simulink model "Praktikum08Gruppe09"  (R2023b)
settings: Solver=VariableStepAuto  StartTime=0.0  StopTime=0.05  RelTol=1e-3
model workspace (MAT data in the model file):
  CodeRate = 0.75
  M = 16
  PunctureVector = [1; 1; 0; 1; 0; 1]
  TracebackDepth = 48
  Trelli.numInputSymbols = 2
  Trelli.numOutputSymbols = 4
  Trelli.numStates = 64
  Trelli.nextStates = [0  32; 0  32; 1  33; 1  33; 2  34; 2  34; 3  35; 3  35; 4  36; 4  36; 5  37; 5  37; 6  38; 6  38; 7  39; 7  39; 8  40; 8  40; 9  41; 9  41; 10  42; 10  42; 11  43; 11  43; 12  44; 12  44; 13  45; 13  45; 14  46; 14  46; 15  47; 15  47; 16  48; 16  48; 17  49; 17  49; 18  50; 18  50; 19  51; 19  51; 20  52; 20  52; 21  53; 21  53; 22  54; 22  54; 23  55; 23  55; 24  56; 24  56; 25  57; 25  57; 26  58; 26  58; 27  59; 27  59; 28  60; 28  60; 29  61; 29  61; 30  62; 30  62; 31  63; 31  63]
  Trelli.outputs = [0  3; 3  0; 1  2; 2  1; 0  3; 3  0; 1  2; 2  1; 3  0; 0  3; 2  1; 1  2; 3  0; 0  3; 2  1; 1  2; 3  0; 0  3; 2  1; 1  2; 3  0; 0  3; 2  1; 1  2; 0  3; 3  0; 1  2; 2  1; 0  3; 3  0; 1  2; 2  1; 2  1; 1  2; 3  0; 0  3; 2  1; 1  2; 3  0; 0  3; 1  2; 2  1; 0  3; 3  0; 1  2; 2  1; 0  3; 3  0; 1  2; 2  1; 0  3; 3  0; 1  2; 2  1; 0  3; 3  0; 2  1; 1  2; 3  0; 0  3; 2  1; 1  2; 3  0; 0  3]
  Ts = 5e-08
undefined symbols (not defined in the file): doppler, get, gray, hot, magnitude
libraries: dspstat3 x10, dspxfrm3 x8, dspobslib x7, commcnvcod2 x6, commdigbbndam3 x6, dspindex x6, commchan3 x4, commrflib2 x4, dspquant2 x4, commsink2 x4, dspsigops x4, commrandsrc3 x2
(part 1 of 2)
settings Model: Creator=suttarar@hu-berlin.de  LastModifiedBy=suttarar@hu-berlin.de

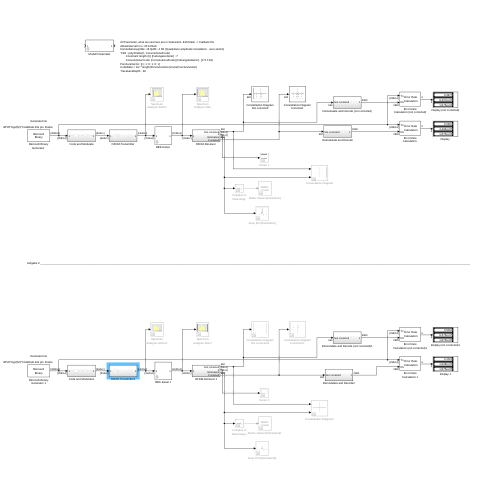
[thumbnail: Simulink's stored preview of the top-level diagram]
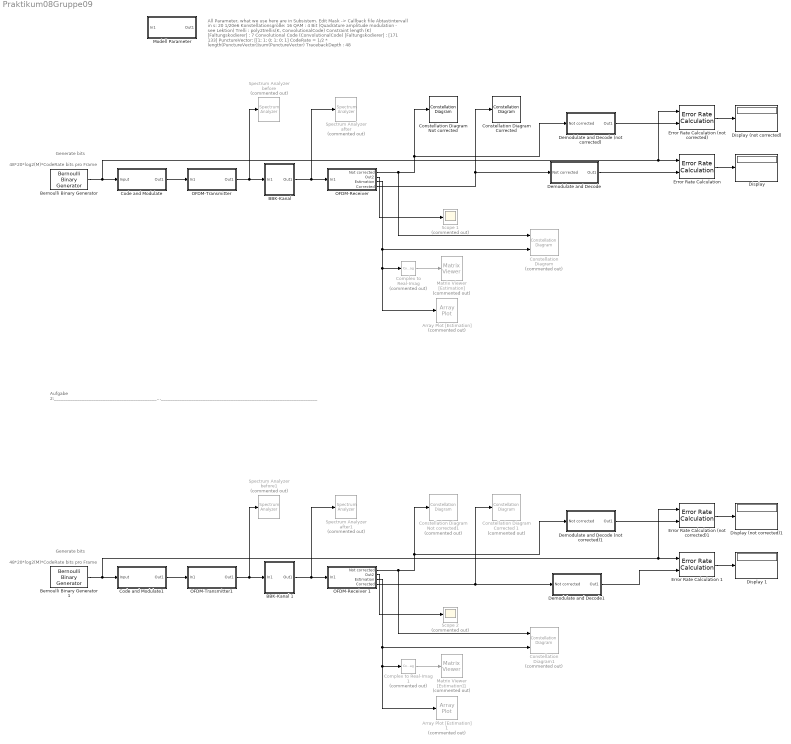
== system Praktikum08Gruppe09 ==
  note: Aufgabe 2:________________________________________________________________________________________________________________________________________________________________________________________________________________________________________________________________________________________
  note: All Parameter, what we use here are in Subsistem. Edit Mask -> Callback file
      | Abtastintervall in s: 20 1/20e6
      | Konstellationsgröße: 16 QAM : 4 Bit (Quadrature amplitude modulation - see Lektion)
      | Trelli : poly2trellis(K, ConvolutionalCode)
      | Constraint length (K) [Faltungskodierer] : 7
      | Convolutional Code (ConvolutionalCode) [Faltungskodierer] : [171 133]
      | PunctureVector: [[1; 1; 0; 1; 0; 1]
      | CodeRate = 1/2 * length(PunctureVector)/sum(PunctureVector)
      | TracebackDepth : 48
  note: 48*20*log2(M)*CodeRate bits pro Frame
  note: Generate bits
  note: 48*20*log2(M)*CodeRate bits pro Frame
  note: Generate bits
  Array Plot [Estimation] : ArrayPlot  Commented=on  WindowPosition=[886.000000,184.000000,800.000000,500.000000,]  ScopeFrameLocation=window  PlotAsMagnitudePhase=on  YLimits=[-0.4803 1.494]
  Array Plot [Estimation]1 : ArrayPlot  Commented=on  WindowPosition=[886.000000,184.000000,800.000000,500.000000,]  ScopeFrameLocation=window  PlotAsMagnitudePhase=on  YLimits=[-0.4803 1.494]
  "BBK-Kanal " : Subsystem  mask{MaxDoppler=20, PathDelays=[0 5 20].*Ts, PathGains=[0 -3 -6], EnableMultipath=1, PathLoss=0, FrequencyOffset=50, PhaseOffset=45, SNR=25}
      mask prompts: MaxDoppler "Dopplerverschiebung"; PathDelays "Pfadverzoergerungen"; PathGains "Pfadverstaerkungen"; EnableMultipath "SwitchBlock"; PathLoss "Pfadverlust"; FrequencyOffset "Frequenzverschiebung"; PhaseOffset "Phasenverschiebung"; SNR "AWG-Rauschen"
  BBK-Kanal 1 : Subsystem  mask{MaxDoppler=20, PathDelays=[0 5 20].*Ts, PathGains=[0 -3 -6], EnableMultipath=1, PathLoss=0, FrequencyOffset=50, PhaseOffset=45, SNR=25}
      mask prompts: MaxDoppler "Dopplerverschiebung"; PathDelays "Pfadverzoergerungen"; PathGains "Pfadverstaerkungen"; EnableMultipath "SwitchBlock"; PathLoss "Pfadverlust"; FrequencyOffset "Frequenzverschiebung"; PhaseOffset "Phasenverschiebung"; SNR "AWG-Rauschen"
  "Bernoulli Binary Generator " : commrandsrc3/Bernoulli Binary Generator  ProbabilityOfZero=0.5  SeedSource=Auto  Seed=0  SampleTime=Ts/(48*20*log2(M)*CodeRate)*64*24  SamplesPerFrame=48*20*log2(M)*CodeRate  OutputDataType=double  SimulateUsing=Interpreted execution
  Bernoulli Binary Generator 1 : commrandsrc3/Bernoulli Binary Generator  ProbabilityOfZero=0.5  SeedSource=Auto  Seed=0  SampleTime=Ts/(48*20*log2(M)*CodeRate)*64*24  SamplesPerFrame=48*20*log2(M)*CodeRate  OutputDataType=double  SimulateUsing=Interpreted execution
  Code and Modulate : Subsystem
  Code and Modulate1 : Subsystem
  "Complex to Real-Imag " : ComplexToRealImag  Commented=on  Output=Real
  Complex to Real-Imag 1 : ComplexToRealImag  Commented=on  Output=Real
  Constellation Diagram : ConstellationDiagram  Commented=on  NumInputPorts=2  WindowPosition=[1234.000000,143.000000,600.000000,600.000000,]  ScopeFrameLocation=window  ReferenceConstellation="{[0.70711+0.70711i        -0.70711+0.70711i        -0.70711-0.70711i         0.70711-0.70711i][0.70711+0.70711i        -0.70711+0.70711i        -0.70711-0.70711i         0.70711-0.70711i]}"  XLimits=[-1.55,1.51]  YLimits=[-1.43,1.46]  ShowLegend=on
  "Constellation Diagram Corrected " : ConstellationDiagram  WindowPosition=[121.000000,289.000000,600.000000,600.000000,]  ScopeFrameLocation=window  ReferenceConstellation="[0.70711+0.70711i        -0.70711+0.70711i        -0.70711-0.70711i         0.70711-0.70711i]"  XLimits=[-1.55,1.51]  YLimits=[-1.43,1.46]  ShowLegend=on
  Constellation Diagram Corrected 1 : ConstellationDiagram  Commented=on  WindowPosition=[121.000000,289.000000,600.000000,600.000000,]  ScopeFrameLocation=window  ReferenceConstellation="[0.70711+0.70711i        -0.70711+0.70711i        -0.70711-0.70711i         0.70711-0.70711i]"  XLimits=[-1.55,1.51]  YLimits=[-1.43,1.46]  ShowLegend=on
  Constellation Diagram Not corrected : ConstellationDiagram  WindowPosition=[922.000000,306.000000,600.000000,600.000000,]  ScopeFrameLocation=window  ReferenceConstellation="[0.70711+0.70711i        -0.70711+0.70711i        -0.70711-0.70711i         0.70711-0.70711i]"  XLimits=[-1.55,1.51]  YLimits=[-1.43,1.46]  ShowLegend=on
  Constellation Diagram Not corrected1 : ConstellationDiagram  Commented=on  WindowPosition=[922.000000,306.000000,600.000000,600.000000,]  ScopeFrameLocation=window  ReferenceConstellation="[0.70711+0.70711i        -0.70711+0.70711i        -0.70711-0.70711i         0.70711-0.70711i]"  XLimits=[-1.55,1.51]  YLimits=[-1.43,1.46]  ShowLegend=on
  Constellation Diagram1 : ConstellationDiagram  Commented=on  NumInputPorts=2  WindowPosition=[1234.000000,143.000000,600.000000,600.000000,]  ScopeFrameLocation=window  ReferenceConstellation="{[0.70711+0.70711i        -0.70711+0.70711i        -0.70711-0.70711i         0.70711-0.70711i][0.70711+0.70711i        -0.70711+0.70711i        -0.70711-0.70711i         0.70711-0.70711i]}"  XLimits=[-1.55,1.51]  YLimits=[-1.43,1.46]  ShowLegend=on
  Demodulate and Decode : Subsystem
  Demodulate and Decode (not corrected) : Subsystem
  Demodulate and Decode (not corrected)1 : Subsystem
  Demodulate and Decode1 : Subsystem
  "Display " : Display
  Display (not corrected) : Display
  Display (not corrected)1 : Display
  Display 1 : Display
  "Error Rate Calculation " : commsink2/Error Rate Calculation  N=TracebackDepth  st_delay=48*20*log2(M)*CodeRate  cp_mode=Entire frame  subframe=[]  PMode=Port  WsName=ErrorVec  RsMode2=off  stop=off  numErr=100  maxBits=1e6
  Error Rate Calculation (not corrected) : commsink2/Error Rate Calculation  N=TracebackDepth  st_delay=48*20*log2(M)*CodeRate  cp_mode=Entire frame  subframe=[]  PMode=Port  WsName=ErrorVec  RsMode2=off  stop=off  numErr=100  maxBits=1e6
  Error Rate Calculation (not corrected)1 : commsink2/Error Rate Calculation  N=TracebackDepth  st_delay=48*20*log2(M)*CodeRate  cp_mode=Entire frame  subframe=[]  PMode=Port  WsName=ErrorVec  RsMode2=off  stop=off  numErr=100  maxBits=1e6
  Error Rate Calculation 1 : commsink2/Error Rate Calculation  N=TracebackDepth  st_delay=48*20*log2(M)*CodeRate  cp_mode=Entire frame  subframe=[]  PMode=Port  WsName=ErrorVec  RsMode2=off  stop=off  numErr=100  maxBits=1e6
  Matrix Viewer [Estimation] : dspobslib/Matrix Viewer  Commented=on  ImageParams=off  CMapStr=gray(256)  AxisColorbar=on  AxisParams=off  AxisOrigin=Upper left corner  AxisTickMode=Auto  XTickRange=[0 1]  YTickRange=[0 1]  XLabel=X-axis  YLabel=Y-axis  ZLabel=Z-axis  FigPos=get(0,'defaultfigureposition')  AxisZoom=off
      settings: YMin=0.99546  YMax=1.0044
  Matrix Viewer [Estimation]1 : dspobslib/Matrix Viewer  Commented=on  ImageParams=off  CMapStr=gray(256)  AxisColorbar=on  AxisParams=off  AxisOrigin=Upper left corner  AxisTickMode=Auto  XTickRange=[0 1]  YTickRange=[0 1]  XLabel=X-axis  YLabel=Y-axis  ZLabel=Z-axis  FigPos=get(0,'defaultfigureposition')  AxisZoom=off
      settings: YMin=0.99546  YMax=1.0044
  Modell Parameter : Subsystem  mask{Ts=1/20e6, M=16, Trelli=poly2trellis(7, [171 133]), PunctureVector=[1; 1; 0; 1; 0; 1], CodeRate=0.75, TracebackDepth=48}
      mask prompts: Ts "Abtastintervall in s"; M "Konstellationsgröße"
  "OFDM-Receiver " : Subsystem
  OFDM-Receiver 1 : Subsystem
  OFDM-Transmitter : Subsystem
  OFDM-Transmitter1 : Subsystem
  Scope 1 : Scope  Commented=on
  Scope 2 : Scope  Commented=on
  Spectrum Analyzer after : SpectrumAnalyzer  Commented=on  WindowPosition=[-15.000000,19.000000,800.000000,500.000000,]  ScopeFrameLocation=window  Span=20000000  StartFrequency=-10000000  StopFrequency=10000000  YLimits=[-31.57647303,17.61555358]
  Spectrum Analyzer after1 : SpectrumAnalyzer  Commented=on  WindowPosition=[-15.000000,19.000000,800.000000,500.000000,]  ScopeFrameLocation=window  Span=20000000  StartFrequency=-10000000  StopFrequency=10000000  YLimits=[-31.57647303,17.61555358]
  Spectrum Analyzer before : SpectrumAnalyzer  Commented=on  WindowPosition=[6.000000,502.000000,800.000000,500.000000,]  ScopeFrameLocation=window  Span=20000000  StartFrequency=-10000000  StopFrequency=10000000  YLimits=[-48.78355479,20.07673212]
  Spectrum Analyzer before1 : SpectrumAnalyzer  Commented=on  WindowPosition=[6.000000,502.000000,800.000000,500.000000,]  ScopeFrameLocation=window  Span=20000000  StartFrequency=-10000000  StopFrequency=10000000  YLimits=[-48.78355479,20.07673212]
  wires:
  Code and Modulate/1(Out1) -> OFDM-Transmitter/1(In1)
  "OFDM-Receiver "/2(Out2) -> Scope 1/1
  "BBK-Kanal "/1(Out1) -> Spectrum Analyzer after/1, "OFDM-Receiver "/1(In1)
  OFDM-Transmitter/1(Out1) -> Spectrum Analyzer before/1, "BBK-Kanal "/1(In1)
  "OFDM-Receiver "/1(Not corrected) -> Demodulate and Decode (not corrected)/1(Not corrected), Constellation Diagram Not corrected/1, Constellation Diagram/1
  "Error Rate Calculation "/1 -> "Display "/1
  "Bernoulli Binary Generator "/1 -> Error Rate Calculation (not corrected)/1, "Error Rate Calculation "/1, Code and Modulate/1(Input)
  "Complex to Real-Imag "/1 -> Matrix Viewer [Estimation]/1
  "OFDM-Receiver "/3(Estimation) -> Constellation Diagram/2, Array Plot [Estimation]/1, "Complex to Real-Imag "/1
  Demodulate and Decode/1(Out1) -> "Error Rate Calculation "/2
  "OFDM-Receiver "/4(Corrected) -> Demodulate and Decode/1(Not corrected), "Constellation Diagram Corrected "/1
  Error Rate Calculation (not corrected)/1 -> Display (not corrected)/1
  Demodulate and Decode (not corrected)/1(Out1) -> Error Rate Calculation (not corrected)/2
  OFDM-Receiver 1/1(Not corrected) -> Demodulate and Decode (not corrected)1/1(Not corrected), Constellation Diagram Not corrected1/1, Constellation Diagram1/1
  Code and Modulate1/1(Out1) -> OFDM-Transmitter1/1(In1)
  Complex to Real-Imag 1/1 -> Matrix Viewer [Estimation]1/1
  BBK-Kanal 1/1(Out1) -> Spectrum Analyzer after1/1, OFDM-Receiver 1/1(In1)
  OFDM-Receiver 1/2(Out2) -> Scope 2/1
  OFDM-Receiver 1/4(Corrected) -> Constellation Diagram Corrected 1/1, Demodulate and Decode1/1(Not corrected)
  Error Rate Calculation 1/1 -> Display 1/1
  Error Rate Calculation (not corrected)1/1 -> Display (not corrected)1/1
  Demodulate and Decode (not corrected)1/1(Out1) -> Error Rate Calculation (not corrected)1/2
  OFDM-Transmitter1/1(Out1) -> Spectrum Analyzer before1/1, BBK-Kanal 1/1(In1)
  Demodulate and Decode1/1(Out1) -> Error Rate Calculation 1/2
  Bernoulli Binary Generator 1/1 -> Error Rate Calculation (not corrected)1/1, Error Rate Calculation 1/1, Code and Modulate1/1(Input)
  OFDM-Receiver 1/3(Estimation) -> Constellation Diagram1/2, Array Plot [Estimation]1/1, Complex to Real-Imag 1/1

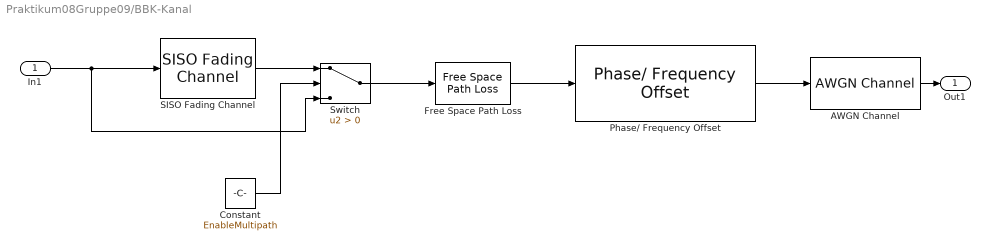
== system Praktikum08Gruppe09/BBK-Kanal  ==
  In1 : Inport
  AWGN Channel : commchan3/AWGN Channel  LegacyMode=off  NoiseMethod="Signal to noise ratio  (SNR)"  noiseMode="Signal to noise ratio  (SNR)"  EbNo=10  EsNo=10  SNR=SNR  BitsPerSymbol=1  SignalPower=1  SamplesPerSymbol=1  SymbolPeriod=1  VarianceSource=Parameter  Variance=1  RandomStream=Global stream  Seed=67  SimulateUsing=Code generation
  Constant : Constant  Value=EnableMultipath
  Free Space Path Loss : commrflib2/Free Space Path Loss  mode=Decibels  dB=PathLoss  d=0.100  fc=1920
  Phase/ Frequency Offset : commrflib2/Phase// Frequency Offset  phaseOffset=PhaseOffset  freqPort=off  freqOffset=FrequencyOffset
      settings: LibrarySourceBlock=|
      | commrfcorlib/Phase//
      | Frequency
      | Offset
  SISO Fading Channel : commchan3/SISO Fading Channel  InheritSampleRate=on  SampleRate=1  PathDelays=PathDelays  AveragePathGains=PathGains  NormalizePathGains=on  FadingDistribution=Rayleigh  KFactor=3  DirectPathDopplerShift=0  DirectPathInitialPhase=0  MaximumDopplerShift=MaxDoppler  DopplerSpectrum=doppler('Jakes')  RandomStream=mt19937ar with seed  Seed=73  PathGainsOutputPort=off  ChannelFilterDelayOutputPort=off  SimulateUsing=Interpreted execution  Visualization=Off  PathsForDopplerDisplay=1  SamplesToDisplay=25%
  Switch : Switch  Criteria=u2 > Threshold  SaturateOnIntegerOverflow=off  InputSameDT=off
  Out1 : Outport
  wires:
  Phase/ Frequency Offset/1 -> AWGN Channel/1
  Free Space Path Loss/1 -> Phase/ Frequency Offset/1
  AWGN Channel/1 -> Out1/1
  Switch/1 -> Free Space Path Loss/1
  SISO Fading Channel/1 -> Switch/1
  In1/1 -> Switch/3, SISO Fading Channel/1
  Constant/1 -> Switch/2

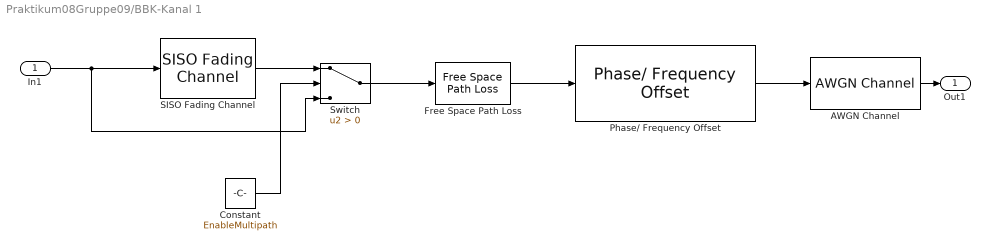
== system Praktikum08Gruppe09/BBK-Kanal 1 ==
  In1 : Inport
  AWGN Channel : commchan3/AWGN Channel  LegacyMode=off  NoiseMethod="Signal to noise ratio  (SNR)"  noiseMode="Signal to noise ratio  (SNR)"  EbNo=10  EsNo=10  SNR=SNR  BitsPerSymbol=1  SignalPower=1  SamplesPerSymbol=1  SymbolPeriod=1  VarianceSource=Parameter  Variance=1  RandomStream=Global stream  Seed=67  SimulateUsing=Code generation
  Constant : Constant  Value=EnableMultipath
  Free Space Path Loss : commrflib2/Free Space Path Loss  mode=Decibels  dB=PathLoss  d=0.100  fc=1920
  Phase/ Frequency Offset : commrflib2/Phase// Frequency Offset  phaseOffset=PhaseOffset  freqPort=off  freqOffset=FrequencyOffset
      settings: LibrarySourceBlock=|
      | commrfcorlib/Phase//
      | Frequency
      | Offset
  SISO Fading Channel : commchan3/SISO Fading Channel  InheritSampleRate=on  SampleRate=1  PathDelays=PathDelays  AveragePathGains=PathGains  NormalizePathGains=on  FadingDistribution=Rayleigh  KFactor=3  DirectPathDopplerShift=0  DirectPathInitialPhase=0  MaximumDopplerShift=MaxDoppler  DopplerSpectrum=doppler('Jakes')  RandomStream=mt19937ar with seed  Seed=73  PathGainsOutputPort=off  ChannelFilterDelayOutputPort=off  SimulateUsing=Interpreted execution  Visualization=Off  PathsForDopplerDisplay=1  SamplesToDisplay=25%
  Switch : Switch  Criteria=u2 > Threshold  SaturateOnIntegerOverflow=off  InputSameDT=off
  Out1 : Outport
  wires:
  Phase/ Frequency Offset/1 -> AWGN Channel/1
  Free Space Path Loss/1 -> Phase/ Frequency Offset/1
  AWGN Channel/1 -> Out1/1
  Switch/1 -> Free Space Path Loss/1
  SISO Fading Channel/1 -> Switch/1
  In1/1 -> Switch/3, SISO Fading Channel/1
  Constant/1 -> Switch/2

== system Praktikum08Gruppe09/Code and Modulate ==
  note: Modulation
  note: Faltungscodierer
  Input : Inport
  "Convolutional Encoder " : commcnvcod2/Convolutional Encoder  trellis=Trelli  opMode=Continuous  DelayedResetAction=off  hasIniStPort=off  hasFinStPort=off  usePuncVector=on  punctureVector=PunctureVector  reset=Unused parameter value
  "Rectangular QAM Modulator Baseband " : commdigbbndam3/Rectangular QAM Modulator Baseband  M=M  InType=Bit  Enc=Gray  Mapping=[0:15]  PowType=Average Power  MinDist=2  AvgPow=1  PeakPow=1  Ph=0  outDtype=double  outWordLen=16  outUDDataType=sfix(16)  outFracLenMode=Best precision  outFracLen=15  outDataTypeStr=double  outLastDataTypeStr=double
  Out1 : Outport
  wires:
  "Convolutional Encoder "/1 -> "Rectangular QAM Modulator Baseband "/1
  "Rectangular QAM Modulator Baseband "/1 -> Out1/1
  Input/1 -> "Convolutional Encoder "/1

== system Praktikum08Gruppe09/Code and Modulate1 ==
  note: Modulation
  note: Faltungscodierer
  Input : Inport
  "Convolutional Encoder " : commcnvcod2/Convolutional Encoder  trellis=Trelli  opMode=Continuous  DelayedResetAction=off  hasIniStPort=off  hasFinStPort=off  usePuncVector=on  punctureVector=PunctureVector  reset=Unused parameter value
  "Rectangular QAM Modulator Baseband " : commdigbbndam3/Rectangular QAM Modulator Baseband  M=M  InType=Bit  Enc=Gray  Mapping=[0:15]  PowType=Average Power  MinDist=2  AvgPow=1  PeakPow=1  Ph=0  outDtype=double  outWordLen=16  outUDDataType=sfix(16)  outFracLenMode=Best precision  outFracLen=15  outDataTypeStr=double  outLastDataTypeStr=double
  Out1 : Outport
  wires:
  "Convolutional Encoder "/1 -> "Rectangular QAM Modulator Baseband "/1
  "Rectangular QAM Modulator Baseband "/1 -> Out1/1
  Input/1 -> "Convolutional Encoder "/1

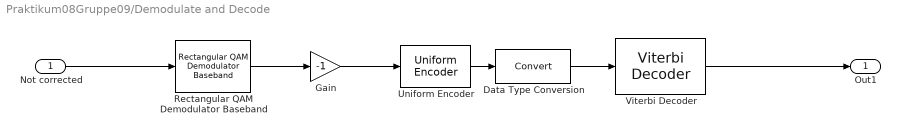
== system Praktikum08Gruppe09/Demodulate and Decode ==
  Not corrected : Inport
  "Data Type Conversion " : DataTypeConversion  SaturateOnIntegerOverflow=off  RndMeth=Floor
  "Gain " : Gain  Gain=-1
  "Rectangular QAM Demodulator Baseband " : commdigbbndam3/Rectangular QAM Demodulator Baseband  M=M  OutType=Bit  DecType=Approximate log-likelihood ratio  VarSource=Dialog  Variance=1  Dec=Gray  Mapping=[0:15]  PowType=Average Power  MinDist=2  AvgPow=1  PeakPow=1  Ph=0  outDtype1=Inherit via internal rule  outDtype2=Inherit via internal rule  derotateFactorWordLen=16  derotateFactorDataTypeStr=Inherit: Same word length as input  derotateFactorLastDataTypeStr=Inherit: Same word length as input  denormFactorWordLen=16  denormFactorDataTypeStr=Inherit: Same word length as input  denormFactorLastDataTypeStr=Inherit: Same word length as input  prodOutWordLen=32  prodOutOverflowMode=Wrap  prodOutRoundingMode=Floor  prodOutOvFlMode=off  prodOutOvFlModeLastStrValue=off  sumWordLen=32
  "Uniform Encoder " : dspquant2/Uniform Encoder  peak=1  bits=4  otype=Unsigned integer
  "Viterbi Decoder " : commcnvcod2/Viterbi Decoder  trellis=Trelli  isPunctured=on  punctureVector=PunctureVector  erasures=off  dectype=Soft decision  nsdecb=4  runSigValErrCheck=off  tbdepth=TracebackDepth  opmode=Continuous  reset=off  delayedResetAction=off  smWordLength=16  outDataType=double
  Out1 : Outport
  wires:
  "Uniform Encoder "/1 -> "Data Type Conversion "/1
  "Gain "/1 -> "Uniform Encoder "/1
  "Data Type Conversion "/1 -> "Viterbi Decoder "/1
  "Rectangular QAM Demodulator Baseband "/1 -> "Gain "/1
  Not corrected/1 -> "Rectangular QAM Demodulator Baseband "/1
  "Viterbi Decoder "/1 -> Out1/1

== system Praktikum08Gruppe09/Demodulate and Decode (not corrected) ==
  Not corrected : Inport
  "Data Type Conversion " : DataTypeConversion  SaturateOnIntegerOverflow=off  RndMeth=Floor
  "Gain " : Gain  Gain=-1
  "Rectangular QAM Demodulator Baseband " : commdigbbndam3/Rectangular QAM Demodulator Baseband  M=M  OutType=Bit  DecType=Approximate log-likelihood ratio  VarSource=Dialog  Variance=1  Dec=Gray  Mapping=[0:15]  PowType=Average Power  MinDist=2  AvgPow=1  PeakPow=1  Ph=0  outDtype1=Inherit via internal rule  outDtype2=Inherit via internal rule  derotateFactorWordLen=16  derotateFactorDataTypeStr=Inherit: Same word length as input  derotateFactorLastDataTypeStr=Inherit: Same word length as input  denormFactorWordLen=16  denormFactorDataTypeStr=Inherit: Same word length as input  denormFactorLastDataTypeStr=Inherit: Same word length as input  prodOutWordLen=32  prodOutOverflowMode=Wrap  prodOutRoundingMode=Floor  prodOutOvFlMode=off  prodOutOvFlModeLastStrValue=off  sumWordLen=32
  "Uniform Encoder " : dspquant2/Uniform Encoder  peak=1  bits=4  otype=Unsigned integer
  "Viterbi Decoder " : commcnvcod2/Viterbi Decoder  trellis=Trelli  isPunctured=on  punctureVector=PunctureVector  erasures=off  dectype=Soft decision  nsdecb=4  runSigValErrCheck=off  tbdepth=TracebackDepth  opmode=Continuous  reset=off  delayedResetAction=off  smWordLength=16  outDataType=double
  Out1 : Outport
  wires:
  "Uniform Encoder "/1 -> "Data Type Conversion "/1
  "Gain "/1 -> "Uniform Encoder "/1
  "Data Type Conversion "/1 -> "Viterbi Decoder "/1
  "Rectangular QAM Demodulator Baseband "/1 -> "Gain "/1
  Not corrected/1 -> "Rectangular QAM Demodulator Baseband "/1
  "Viterbi Decoder "/1 -> Out1/1

== system Praktikum08Gruppe09/Demodulate and Decode (not corrected)1 ==
  Not corrected : Inport
  "Data Type Conversion " : DataTypeConversion  SaturateOnIntegerOverflow=off  RndMeth=Floor
  "Gain " : Gain  Gain=-1
  "Rectangular QAM Demodulator Baseband " : commdigbbndam3/Rectangular QAM Demodulator Baseband  M=M  OutType=Bit  DecType=Approximate log-likelihood ratio  VarSource=Dialog  Variance=1  Dec=Gray  Mapping=[0:15]  PowType=Average Power  MinDist=2  AvgPow=1  PeakPow=1  Ph=0  outDtype1=Inherit via internal rule  outDtype2=Inherit via internal rule  derotateFactorWordLen=16  derotateFactorDataTypeStr=Inherit: Same word length as input  derotateFactorLastDataTypeStr=Inherit: Same word length as input  denormFactorWordLen=16  denormFactorDataTypeStr=Inherit: Same word length as input  denormFactorLastDataTypeStr=Inherit: Same word length as input  prodOutWordLen=32  prodOutOverflowMode=Wrap  prodOutRoundingMode=Floor  prodOutOvFlMode=off  prodOutOvFlModeLastStrValue=off  sumWordLen=32
  "Uniform Encoder " : dspquant2/Uniform Encoder  peak=1  bits=4  otype=Unsigned integer
  "Viterbi Decoder " : commcnvcod2/Viterbi Decoder  trellis=Trelli  isPunctured=on  punctureVector=PunctureVector  erasures=off  dectype=Soft decision  nsdecb=4  runSigValErrCheck=off  tbdepth=TracebackDepth  opmode=Continuous  reset=off  delayedResetAction=off  smWordLength=16  outDataType=double
  Out1 : Outport
  wires:
  "Uniform Encoder "/1 -> "Data Type Conversion "/1
  "Gain "/1 -> "Uniform Encoder "/1
  "Data Type Conversion "/1 -> "Viterbi Decoder "/1
  "Rectangular QAM Demodulator Baseband "/1 -> "Gain "/1
  Not corrected/1 -> "Rectangular QAM Demodulator Baseband "/1
  "Viterbi Decoder "/1 -> Out1/1

== system Praktikum08Gruppe09/Demodulate and Decode1 ==
  Not corrected : Inport
  "Data Type Conversion " : DataTypeConversion  SaturateOnIntegerOverflow=off  RndMeth=Floor
  "Gain " : Gain  Gain=-1
  "Rectangular QAM Demodulator Baseband " : commdigbbndam3/Rectangular QAM Demodulator Baseband  M=M  OutType=Bit  DecType=Approximate log-likelihood ratio  VarSource=Dialog  Variance=1  Dec=Gray  Mapping=[0:15]  PowType=Average Power  MinDist=2  AvgPow=1  PeakPow=1  Ph=0  outDtype1=Inherit via internal rule  outDtype2=Inherit via internal rule  derotateFactorWordLen=16  derotateFactorDataTypeStr=Inherit: Same word length as input  derotateFactorLastDataTypeStr=Inherit: Same word length as input  denormFactorWordLen=16  denormFactorDataTypeStr=Inherit: Same word length as input  denormFactorLastDataTypeStr=Inherit: Same word length as input  prodOutWordLen=32  prodOutOverflowMode=Wrap  prodOutRoundingMode=Floor  prodOutOvFlMode=off  prodOutOvFlModeLastStrValue=off  sumWordLen=32
  "Uniform Encoder " : dspquant2/Uniform Encoder  peak=1  bits=4  otype=Unsigned integer
  "Viterbi Decoder " : commcnvcod2/Viterbi Decoder  trellis=Trelli  isPunctured=on  punctureVector=PunctureVector  erasures=off  dectype=Soft decision  nsdecb=4  runSigValErrCheck=off  tbdepth=TracebackDepth  opmode=Continuous  reset=off  delayedResetAction=off  smWordLength=16  outDataType=double
  Out1 : Outport
  wires:
  "Uniform Encoder "/1 -> "Data Type Conversion "/1
  "Gain "/1 -> "Uniform Encoder "/1
  "Data Type Conversion "/1 -> "Viterbi Decoder "/1
  "Rectangular QAM Demodulator Baseband "/1 -> "Gain "/1
  Not corrected/1 -> "Rectangular QAM Demodulator Baseband "/1
  "Viterbi Decoder "/1 -> Out1/1

== system Praktikum08Gruppe09/Modell Parameter ==
  In1 : Inport
  Out1 : Outport
  wires:
  In1/1 -> Out1/1

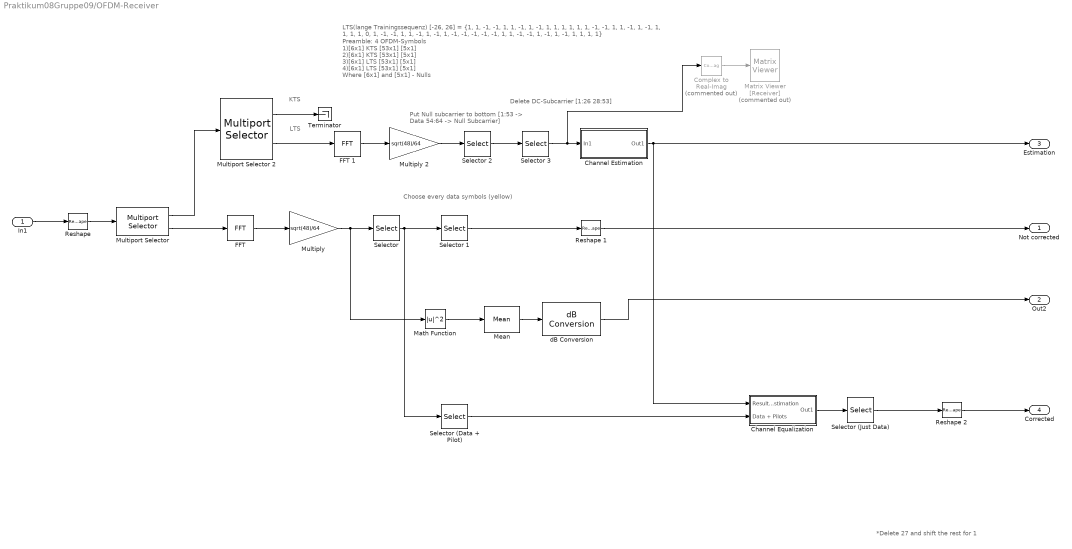
== system Praktikum08Gruppe09/OFDM-Receiver  ==
  note: *Delete 27 and shift the rest for 1
  note: Delete DC-Subcarrier [1:26 28:53]
  note: Put Null subcarrier to bottom
      | [1:53 -> Data 54:64 -> Null Subcarrier]
  note: LTS
  note: KTS
  note: Choose every data symbols (yellow)
  note: LTS(lange Trainingssequenz) [-26, 26] = {1, 1, -1, -1, 1, 1, -1, 1, -1, 1, 1, 1, 1, 1, 1, -1, -1, 1, 1, -1, 1, -1, 1, 1, 1, 1, 0, 1, -1, -1, 1, 1, -1, 1, -1, 1, -1, -1, -1, -1, -1, 1, 1, -1, -1, 1, -1, 1, -1, 1, 1, 1, 1}
  note: Preamble: 4 OFDM-Symbols
      | 1)[6x1] KTS [53x1] [5x1]
      | 2)[6x1] KTS [53x1] [5x1]
      | 3)[6x1] LTS [53x1] [5x1]
      | 4)[6x1] LTS [53x1] [5x1]
      |
      | Where [6x1] and [5x1] - Nulls
  In1 : Inport
  Channel Equalization : Subsystem
  Channel Estimation : Subsystem
  "Complex to Real-Imag " : ComplexToRealImag  Commented=on  Output=Real
  "FFT " : dspxfrm3/FFT  FFTImplementation=Auto  CompMethod=Table lookup  TableOpt=NEW  TableOptActive=Speed  BitRevOrder=off  Normalize=off  InheritFFTLength=on  FFTLength=64  WrapInput=on  roundingMode=Floor  overflowMode=off  firstCoeffDataTypeStr=Inherit: Same word length as input  firstCoeffLastDataTypeStr=Inherit: Same word length as input  outputMin=[]  outputMax=[]
  FFT 1 : dspxfrm3/FFT  FFTImplementation=Auto  CompMethod=Table lookup  TableOpt=NEW  TableOptActive=Speed  BitRevOrder=off  Normalize=off  InheritFFTLength=on  FFTLength=64  WrapInput=on  roundingMode=Floor  overflowMode=off  firstCoeffDataTypeStr=Inherit: Same word length as input  firstCoeffLastDataTypeStr=Inherit: Same word length as input  outputMin=[]  outputMax=[]
  "Math Function " : Math  Operator=magnitude^2
  Matrix Viewer [Receiver] : dspobslib/Matrix Viewer  Commented=on  ImageParams=off  CMapStr=gray(256)  AxisColorbar=on  AxisParams=off  AxisOrigin=Upper left corner  AxisTickMode=Auto  XTickRange=[0 1]  YTickRange=[0 1]  XLabel=X-axis  YLabel=Y-axis  ZLabel=Z-axis  FigPos=get(0,'defaultfigureposition')  AxisZoom=off
      settings: YMin=-1.0038  YMax=1.0044
  "Mean " : dspstat3/Mean  run=off  InputProcessing=Columns as channels (frame based)  reset_popup=None  directionMode=Each row  dimension=1  roiEnable=off  roiType=Rectangles  roiPortion=Entire ROI  roiOutput=Individual statistics for each ROI  roiFlag=off  roundingMode=Floor  overflowMode=off  outputDataTypeStr=Inherit: Same as accumulator  outputMin=[]  outputMax=[]  outputLastDataTypeStr=Inherit: Same as accumulator
  "Multiply " : Gain  Gain=sqrt(48)/64
  Multiply 2 : Gain  Gain=sqrt(48)/64
  "Multiport Selector " : dspindex/Multiport Selector  rowsOrCols=Columns  idxCellArray={[1:4], [5:24]}  idxErrMode=Clip Index
  Multiport Selector 2 : dspindex/Multiport Selector  rowsOrCols=Columns  idxCellArray={[1:2], [3:4]}  idxErrMode=Clip Index
  "Reshape " : Reshape  OutputDimensionality=Customize  OutputDimensions=[64,24]
  Reshape 1 : Reshape  OutputDimensions=[64,24]
  Reshape 2 : Reshape  OutputDimensions=[64,24]
  "Selector " : Selector  NumberOfDimensions=2  InputPortWidth=3  IndexOptions=Index vector (dialog),Select all  Indices=[39:64 1:38],1  OutputSizes=1,1
  Selector (Data + Pilot) : Selector  NumberOfDimensions=2  InputPortWidth=3  IndexOptions=Index vector (dialog),Select all  Indices=[1:26 28:53],1  OutputSizes=1,1
  Selector (Just Data) : Selector  NumberOfDimensions=2  InputPortWidth=3  IndexOptions=Index vector (dialog),Select all  Indices=[1:5 7:19 21:32 34:46 48:52],1  OutputSizes=1,1
  Selector 1 : Selector  NumberOfDimensions=2  InputPortWidth=3  IndexOptions=Index vector (dialog),Select all  Indices=[1:5 7:19 21:26 28:33 35:47 49:53],1  OutputSizes=1,1
  Selector 2 : Selector  NumberOfDimensions=2  InputPortWidth=3  IndexOptions=Index vector (dialog),Select all  Indices=[39:64 1:38],1  OutputSizes=1,1
  Selector 3 : Selector  NumberOfDimensions=2  InputPortWidth=3  IndexOptions=Index vector (dialog),Select all  Indices=[1:26 28:53],1  OutputSizes=1,1
  "Terminator " : Terminator
  "dB Conversion " : dspmathops/dB Conversion  dBtype=dB  intype=Power  R=1  fuzz=off
      settings: LibrarySourceBlock=commutil2/dB Conversion
  Not corrected : Outport
  Out2 : Outport  Port=2
  Estimation : Outport  Port=3
  Corrected : Outport  Port=4
  wires:
  "Mean "/1 -> "dB Conversion "/1
  "Math Function "/1 -> "Mean "/1
  "FFT "/1 -> "Multiply "/1
  In1/1 -> "Reshape "/1
  "Selector "/1 -> Selector (Data + Pilot)/1, Selector 1/1
  "Reshape "/1 -> "Multiport Selector "/1
  "Multiport Selector "/2 -> "FFT "/1
  "Multiport Selector "/1 -> Multiport Selector 2/1
  "dB Conversion "/1 -> Out2/1
  Selector 1/1 -> Reshape 1/1
  Reshape 1/1 -> Not corrected/1
  "Multiply "/1 -> "Math Function "/1, "Selector "/1
  Multiport Selector 2/1 -> "Terminator "/1
  Multiport Selector 2/2 -> FFT 1/1
  Channel Estimation/1(Out1) -> Channel Equalization/1(Result from Channel Estimation), Estimation/1
  Selector 2/1 -> Selector 3/1
  Multiply 2/1 -> Selector 2/1
  FFT 1/1 -> Multiply 2/1
  Selector 3/1 -> "Complex to Real-Imag "/1, Channel Estimation/1(In1)
  "Complex to Real-Imag "/1 -> Matrix Viewer [Receiver]/1
  Selector (Data + Pilot)/1 -> Channel Equalization/2(Data + Pilots)
  Channel Equalization/1(Out1) -> Selector (Just Data)/1
  Selector (Just Data)/1 -> Reshape 2/1
  Reshape 2/1 -> Corrected/1

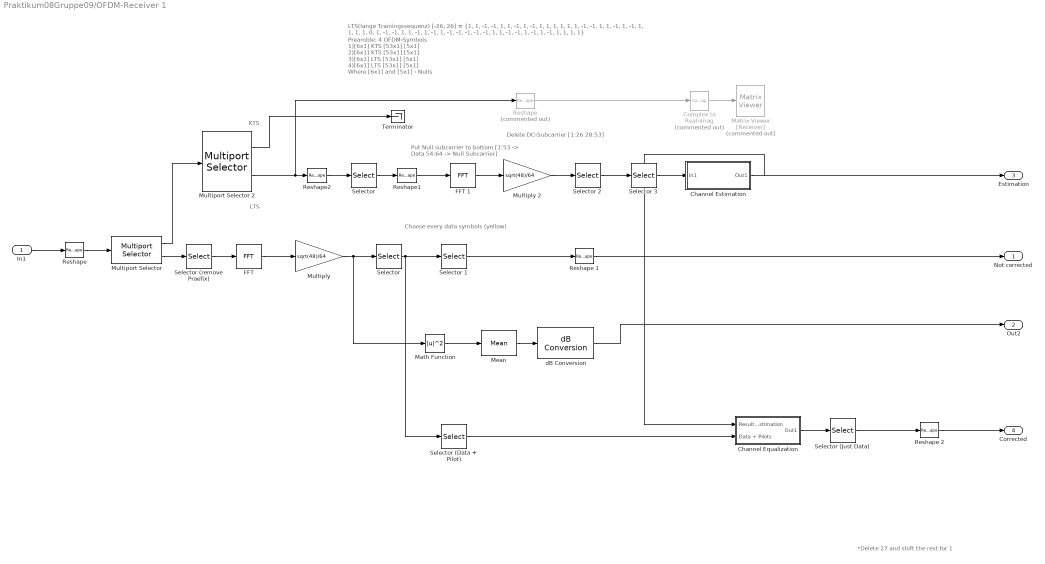
== system Praktikum08Gruppe09/OFDM-Receiver 1 ==
  note: *Delete 27 and shift the rest for 1
  note: Delete DC-Subcarrier [1:26 28:53]
  note: Put Null subcarrier to bottom
      | [1:53 -> Data 54:64 -> Null Subcarrier]
  note: LTS
  note: KTS
  note: Choose every data symbols (yellow)
  note: LTS(lange Trainingssequenz) [-26, 26] = {1, 1, -1, -1, 1, 1, -1, 1, -1, 1, 1, 1, 1, 1, 1, -1, -1, 1, 1, -1, 1, -1, 1, 1, 1, 1, 0, 1, -1, -1, 1, 1, -1, 1, -1, 1, -1, -1, -1, -1, -1, 1, 1, -1, -1, 1, -1, 1, -1, 1, 1, 1, 1}
  note: Preamble: 4 OFDM-Symbols
      | 1)[6x1] KTS [53x1] [5x1]
      | 2)[6x1] KTS [53x1] [5x1]
      | 3)[6x1] LTS [53x1] [5x1]
      | 4)[6x1] LTS [53x1] [5x1]
      |
      | Where [6x1] and [5x1] - Nulls
  In1 : Inport
  Channel Equalization : Subsystem
  Channel Estimation : Subsystem
  "Complex to Real-Imag " : ComplexToRealImag  Commented=on  Output=Real
  "FFT " : dspxfrm3/FFT  FFTImplementation=Auto  CompMethod=Table lookup  TableOpt=NEW  TableOptActive=Speed  BitRevOrder=off  Normalize=off  InheritFFTLength=on  FFTLength=64  WrapInput=on  roundingMode=Floor  overflowMode=off  firstCoeffDataTypeStr=Inherit: Same word length as input  firstCoeffLastDataTypeStr=Inherit: Same word length as input  outputMin=[]  outputMax=[]
  FFT 1 : dspxfrm3/FFT  FFTImplementation=Auto  CompMethod=Table lookup  TableOpt=NEW  TableOptActive=Speed  BitRevOrder=off  Normalize=off  InheritFFTLength=on  FFTLength=64  WrapInput=on  roundingMode=Floor  overflowMode=off  firstCoeffDataTypeStr=Inherit: Same word length as input  firstCoeffLastDataTypeStr=Inherit: Same word length as input  outputMin=[]  outputMax=[]
  "Math Function " : Math  Operator=magnitude^2
  Matrix Viewer [Receiver] : dspobslib/Matrix Viewer  Commented=on  ImageParams=off  CMapStr=gray(256)  AxisColorbar=on  AxisParams=off  AxisOrigin=Upper left corner  AxisTickMode=Auto  XTickRange=[0 1]  YTickRange=[0 1]  XLabel=X-axis  YLabel=Y-axis  ZLabel=Z-axis  FigPos=get(0,'defaultfigureposition')  AxisZoom=off
      settings: YMin=-1.4434  YMax=1.4434
  "Mean " : dspstat3/Mean  run=off  InputProcessing=Columns as channels (frame based)  reset_popup=None  directionMode=Each row  dimension=1  roiEnable=off  roiType=Rectangles  roiPortion=Entire ROI  roiOutput=Individual statistics for each ROI  roiFlag=off  roundingMode=Floor  overflowMode=off  outputDataTypeStr=Inherit: Same as accumulator  outputMin=[]  outputMax=[]  outputLastDataTypeStr=Inherit: Same as accumulator
  "Multiply " : Gain  Gain=sqrt(48)/64
  Multiply 2 : Gain  Gain=sqrt(48)/64
  "Multiport Selector " : dspindex/Multiport Selector  rowsOrCols=Columns  idxCellArray={[1:4], [5:24]}  idxErrMode=Clip Index
  Multiport Selector 2 : dspindex/Multiport Selector  rowsOrCols=Columns  idxCellArray={[1:2], [3:4]}  idxErrMode=Clip Index
  Reshape : Reshape  Commented=on  OutputDimensionality=Column vector (2-D)
  "Reshape " : Reshape  OutputDimensionality=Customize  OutputDimensions=[80,24]
  Reshape 1 : Reshape  OutputDimensions=[64,24]
  Reshape 2 : Reshape  OutputDimensions=[64,24]
  Reshape1 : Reshape  OutputDimensionality=Customize  OutputDimensions=[64,2]
  Reshape2 : Reshape  OutputDimensionality=Column vector (2-D)
  Selector : Selector  NumberOfDimensions=2  InputPortWidth=3  IndexOptions=Index vector (dialog),Select all  Indices=[33:160],1  OutputSizes=1,1
  "Selector " : Selector  NumberOfDimensions=2  InputPortWidth=3  IndexOptions=Index vector (dialog),Select all  Indices=[39:64 1:38],1  OutputSizes=1,1
  Selector (remove Praefix) : Selector  NumberOfDimensions=2  InputPortWidth=3  IndexOptions=Index vector (dialog),Select all  Indices=[17:80],1  OutputSizes=1,1
  Selector (Data + Pilot) : Selector  NumberOfDimensions=2  InputPortWidth=3  IndexOptions=Index vector (dialog),Select all  Indices=[1:26 28:53],1  OutputSizes=1,1
  Selector (Just Data) : Selector  NumberOfDimensions=2  InputPortWidth=3  IndexOptions=Index vector (dialog),Select all  Indices=[1:5 7:19 21:32 34:46 48:52],1  OutputSizes=1,1
  Selector 1 : Selector  NumberOfDimensions=2  InputPortWidth=3  IndexOptions=Index vector (dialog),Select all  Indices=[1:5 7:19 21:26 28:33 35:47 49:53],1  OutputSizes=1,1
  Selector 2 : Selector  NumberOfDimensions=2  InputPortWidth=3  IndexOptions=Index vector (dialog),Select all  Indices=[39:64 1:38],1  OutputSizes=1,1
  Selector 3 : Selector  NumberOfDimensions=2  InputPortWidth=3  IndexOptions=Index vector (dialog),Select all  Indices=[1:26 28:53],1  OutputSizes=1,1
  "Terminator " : Terminator
  "dB Conversion " : dspmathops/dB Conversion  dBtype=dB  intype=Power  R=1  fuzz=off
      settings: LibrarySourceBlock=commutil2/dB Conversion
  Not corrected : Outport
  Out2 : Outport  Port=2
  Estimation : Outport  Port=3
  Corrected : Outport  Port=4
  wires:
  "Mean "/1 -> "dB Conversion "/1
  "Math Function "/1 -> "Mean "/1
  "FFT "/1 -> "Multiply "/1
  In1/1 -> "Reshape "/1
  "Selector "/1 -> Selector (Data + Pilot)/1, Selector 1/1
  "Reshape "/1 -> "Multiport Selector "/1
  "Multiport Selector "/2 -> Selector (remove Praefix)/1
  "Multiport Selector "/1 -> Multiport Selector 2/1
  "dB Conversion "/1 -> Out2/1
  Selector 1/1 -> Reshape 1/1
  Reshape 1/1 -> Not corrected/1
  "Multiply "/1 -> "Math Function "/1, "Selector "/1
  Channel Estimation/1(Out1) -> Channel Equalization/1(Result from Channel Estimation), Estimation/1
  Selector 2/1 -> Selector 3/1
  Multiply 2/1 -> Selector 2/1
  FFT 1/1 -> Multiply 2/1
  Selector 3/1 -> Channel Estimation/1(In1)
  "Complex to Real-Imag "/1 -> Matrix Viewer [Receiver]/1
  Selector (Data + Pilot)/1 -> Channel Equalization/2(Data + Pilots)
  Channel Equalization/1(Out1) -> Selector (Just Data)/1
  Selector (Just Data)/1 -> Reshape 2/1
  Reshape 2/1 -> Corrected/1
  Selector (remove Praefix)/1 -> "FFT "/1
  Multiport Selector 2/2 -> Reshape/1, Reshape2/1
  Multiport Selector 2/1 -> "Terminator "/1
  Reshape/1 -> "Complex to Real-Imag "/1
  Selector/1 -> Reshape1/1
  Reshape1/1 -> FFT 1/1
  Reshape2/1 -> Selector/1

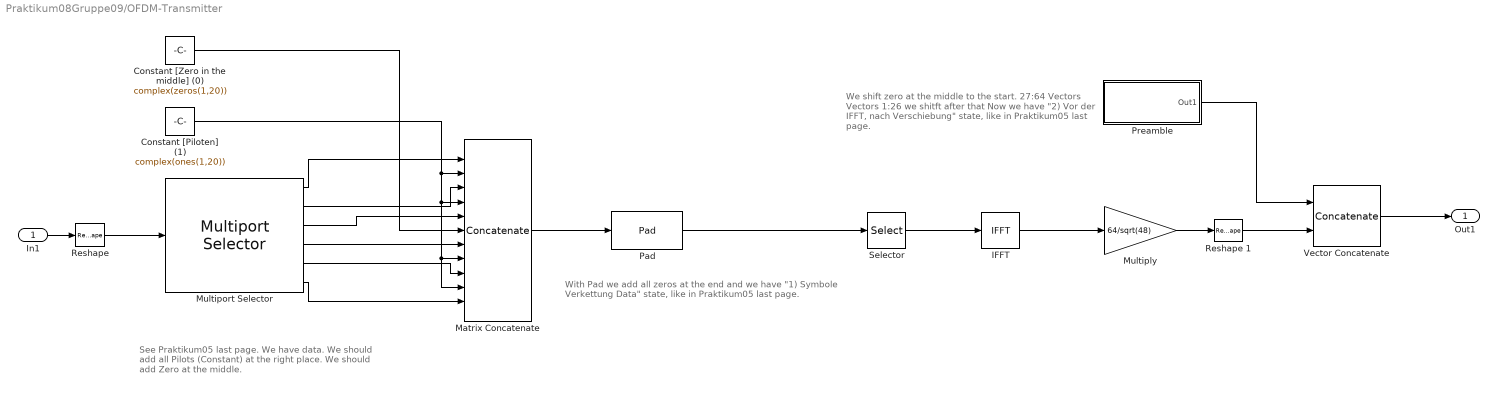
== system Praktikum08Gruppe09/OFDM-Transmitter ==
  note: With Pad we add all zeros at the end and we have
      | "1) Symbole Verkettung Data" state, like in Praktikum05 last page.
  note: See Praktikum05 last page. We have data.
      | We should add all Pilots (Constant) at the right place.
      | We should add Zero at the middle.
  note: We shift zero at the middle to the start.
      | 27:64 Vectors
      | Vectors 1:26 we shitft after that
      | Now we have "2) Vor der IFFT,
      | nach Verschiebung" state, like in Praktikum05 last page.
  In1 : Inport
  Constant [Piloten] (1) : Constant  Value=complex(ones(1,20))  VectorParams1D=off
  Constant [Zero in the middle] (0) : Constant  Value=complex(zeros(1,20))  VectorParams1D=off
  "IFFT " : dspxfrm3/IFFT  FFTImplementation=Auto  CompMethod=Table lookup  TableOpt=NEW  TableOptActive=Speed  BitRevOrder=off  cs_in=off  Normalize=on  InheritFFTLength=on  FFTLength=64  WrapInput=on  mode=Complex  outSamplingMode=Sample based  roundingMode=Floor  overflowMode=off  firstCoeffDataTypeStr=Inherit: Same word length as input  firstCoeffLastDataTypeStr=Inherit: Same word length as input  outputMin=[]  outputMax=[]
  "Matrix Concatenate " : Concatenate  NumInputs=11  Mode=Multidimensional array
  "Multiply " : Gain  Gain=64/sqrt(48)
  Multiport Selector : dspindex/Multiport Selector  rowsOrCols=Rows  idxCellArray={[1:5], [6:18], [19:24], [25:30], [31:43], [44:48]}  idxErrMode=Clip Index
      settings: LibrarySourceBlock=|
      | dsphdlsupportsigmgmt/Multiport
      | Selector
  "Pad " : dspsigops/Pad  padAlong=Columns  dimsToPad=1  valSrc=Specify via dialog  padVal=0  spec=Output size  padNumOutRowsSpecMethod=User-specified  numOutRows=64  padNumOutColsSpecMethod=User-specified  numOutCols=1  isVarDimsMode=off  padBeginning=0  padEnd=0  outSizeMode=User-specified  outSize=1  padSigAt=End  trunc_flag=None  roundingMode=Floor  overflowMode=off  truncOrWrapMode=Truncate  wrap_flag=None
  Preamble : Subsystem
  "Reshape " : Reshape  OutputDimensionality=Customize  OutputDimensions=[48,20]
  Reshape 1 : Reshape  OutputDimensionality=Column vector (2-D)  OutputDimensions=[64,24]
  "Selector " : Selector  NumberOfDimensions=2  InputPortWidth=3  IndexOptions=Index vector (dialog),Select all  Indices=[27:64 1:26],1  OutputSizes=1,1
  "Vector Concatenate " : Concatenate
  Out1 : Outport
  wires:
  In1/1 -> "Reshape "/1
  "Reshape "/1 -> Multiport Selector/1
  "Pad "/1 -> "Selector "/1
  "Matrix Concatenate "/1 -> "Pad "/1
  Multiport Selector/1 -> "Matrix Concatenate "/1
  Multiport Selector/2 -> "Matrix Concatenate "/3
  Multiport Selector/3 -> "Matrix Concatenate "/5
  Multiport Selector/4 -> "Matrix Concatenate "/7
  Multiport Selector/5 -> "Matrix Concatenate "/9
  Multiport Selector/6 -> "Matrix Concatenate "/11
  Constant [Piloten] (1)/1 -> "Matrix Concatenate "/10, "Matrix Concatenate "/8, "Matrix Concatenate "/4, "Matrix Concatenate "/2
  Constant [Zero in the middle] (0)/1 -> "Matrix Concatenate "/6
  "Selector "/1 -> "IFFT "/1
  "IFFT "/1 -> "Multiply "/1
  "Multiply "/1 -> Reshape 1/1
  Reshape 1/1 -> "Vector Concatenate "/2
  "Vector Concatenate "/1 -> Out1/1
  Preamble/1(Out1) -> "Vector Concatenate "/1

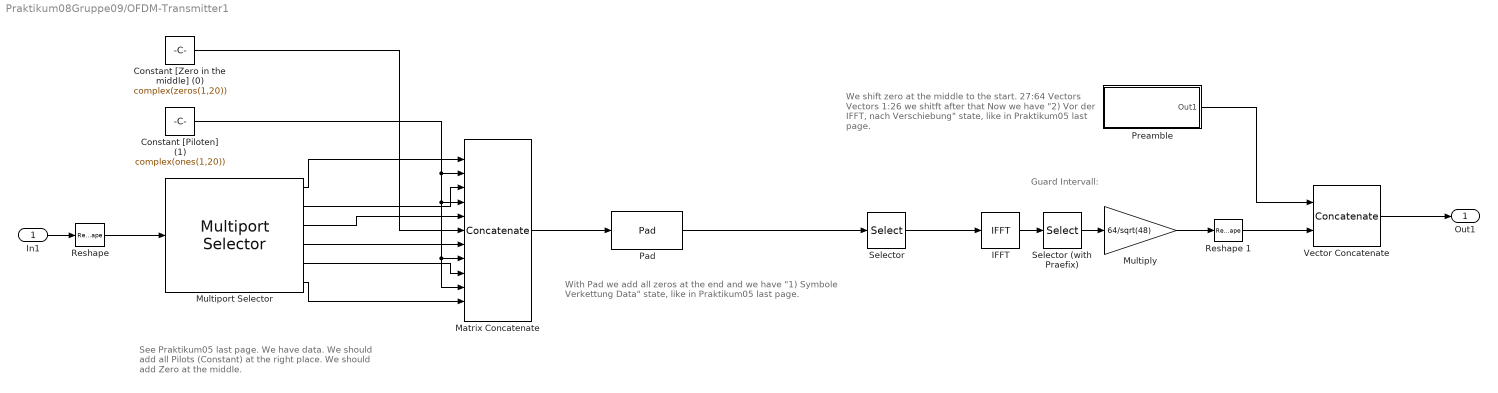
== system Praktikum08Gruppe09/OFDM-Transmitter1 ==
  note: Guard Intervall:
  note: With Pad we add all zeros at the end and we have
      | "1) Symbole Verkettung Data" state, like in Praktikum05 last page.
  note: See Praktikum05 last page. We have data.
      | We should add all Pilots (Constant) at the right place.
      | We should add Zero at the middle.
  note: We shift zero at the middle to the start.
      | 27:64 Vectors
      | Vectors 1:26 we shitft after that
      | Now we have "2) Vor der IFFT,
      | nach Verschiebung" state, like in Praktikum05 last page.
  In1 : Inport
  Constant [Piloten] (1) : Constant  Value=complex(ones(1,20))  VectorParams1D=off
  Constant [Zero in the middle] (0) : Constant  Value=complex(zeros(1,20))  VectorParams1D=off
  "IFFT " : dspxfrm3/IFFT  FFTImplementation=Auto  CompMethod=Table lookup  TableOpt=NEW  TableOptActive=Speed  BitRevOrder=off  cs_in=off  Normalize=on  InheritFFTLength=on  FFTLength=64  WrapInput=on  mode=Complex  outSamplingMode=Sample based  roundingMode=Floor  overflowMode=off  firstCoeffDataTypeStr=Inherit: Same word length as input  firstCoeffLastDataTypeStr=Inherit: Same word length as input  outputMin=[]  outputMax=[]
  "Matrix Concatenate " : Concatenate  NumInputs=11  Mode=Multidimensional array
  "Multiply " : Gain  Gain=64/sqrt(48)
  Multiport Selector : dspindex/Multiport Selector  rowsOrCols=Rows  idxCellArray={[1:5], [6:18], [19:24], [25:30], [31:43], [44:48]}  idxErrMode=Clip Index
      settings: LibrarySourceBlock=|
      | dsphdlsupportsigmgmt/Multiport
      | Selector
  "Pad " : dspsigops/Pad  padAlong=Columns  dimsToPad=1  valSrc=Specify via dialog  padVal=0  spec=Output size  padNumOutRowsSpecMethod=User-specified  numOutRows=64  padNumOutColsSpecMethod=User-specified  numOutCols=1  isVarDimsMode=off  padBeginning=0  padEnd=0  outSizeMode=User-specified  outSize=1  padSigAt=End  trunc_flag=None  roundingMode=Floor  overflowMode=off  truncOrWrapMode=Truncate  wrap_flag=None
  Preamble : Subsystem
  "Reshape " : Reshape  OutputDimensionality=Customize  OutputDimensions=[48,20]
  Reshape 1 : Reshape  OutputDimensionality=Column vector (2-D)  OutputDimensions=[64,24]
  "Selector " : Selector  NumberOfDimensions=2  InputPortWidth=3  IndexOptions=Index vector (dialog),Select all  Indices=[27:64 1:26],1  OutputSizes=1,1
  Selector (with Praefix) : Selector  NumberOfDimensions=2  InputPortWidth=3  IndexOptions=Index vector (dialog),Select all  Indices=[49:64, 1:64],1  OutputSizes=1,1
  "Vector Concatenate " : Concatenate
  Out1 : Outport
  wires:
  In1/1 -> "Reshape "/1
  "Reshape "/1 -> Multiport Selector/1
  "Pad "/1 -> "Selector "/1
  "Matrix Concatenate "/1 -> "Pad "/1
  Multiport Selector/1 -> "Matrix Concatenate "/1
  Multiport Selector/2 -> "Matrix Concatenate "/3
  Multiport Selector/3 -> "Matrix Concatenate "/5
  Multiport Selector/4 -> "Matrix Concatenate "/7
  Multiport Selector/5 -> "Matrix Concatenate "/9
  Multiport Selector/6 -> "Matrix Concatenate "/11
  Constant [Piloten] (1)/1 -> "Matrix Concatenate "/10, "Matrix Concatenate "/8, "Matrix Concatenate "/4, "Matrix Concatenate "/2
  Constant [Zero in the middle] (0)/1 -> "Matrix Concatenate "/6
  "Selector "/1 -> "IFFT "/1
  "IFFT "/1 -> Selector (with Praefix)/1
  "Multiply "/1 -> Reshape 1/1
  Reshape 1/1 -> "Vector Concatenate "/2
  "Vector Concatenate "/1 -> Out1/1
  Preamble/1(Out1) -> "Vector Concatenate "/1
  Selector (with Praefix)/1 -> "Multiply "/1

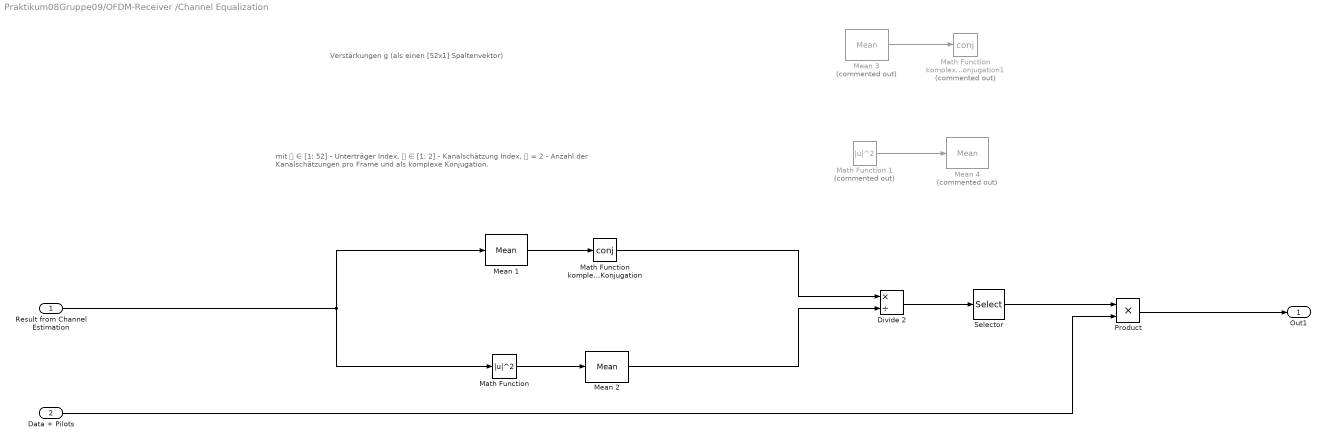
== system Praktikum08Gruppe09/OFDM-Receiver /Channel Equalization ==
  note: mit 𝑢 ∈ [1: 52] - Unterträger Index, 𝑛 ∈ [1: 2] - Kanalschätzung Index, 𝑁 = 2 - Anzahl der Kanalschätzungen pro Frame und als komplexe Konjugation.
  note: Verstärkungen g (als einen [52x1] Spaltenvektor)
  Result from Channel Estimation : Inport
  Data + Pilots : Inport  Port=2
  Divide 2 : Product  Inputs=*/
  "Math Function " : Math  Operator=magnitude^2
  Math Function 1 : Math  Commented=on  Operator=magnitude^2
  Math Function komplexe Konjugation : Math  Operator=conj  OutputSignalType=complex
  Math Function komplexe Konjugation1 : Math  Commented=on  Operator=conj  OutputSignalType=complex
  Mean 1 : dspstat3/Mean  run=off  InputProcessing=Columns as channels (frame based)  reset_popup=None  directionMode=Each row  dimension=1  roiEnable=off  roiType=Rectangles  roiPortion=Entire ROI  roiOutput=Individual statistics for each ROI  roiFlag=off  roundingMode=Floor  overflowMode=off  outputDataTypeStr=Inherit: Same as accumulator  outputMin=[]  outputMax=[]  outputLastDataTypeStr=Inherit: Same as accumulator
  Mean 2 : dspstat3/Mean  run=off  InputProcessing=Columns as channels (frame based)  reset_popup=None  directionMode=Each row  dimension=1  roiEnable=off  roiType=Rectangles  roiPortion=Entire ROI  roiOutput=Individual statistics for each ROI  roiFlag=off  roundingMode=Floor  overflowMode=off  outputDataTypeStr=Inherit: Same as accumulator  outputMin=[]  outputMax=[]  outputLastDataTypeStr=Inherit: Same as accumulator
  Mean 3 : dspstat3/Mean  Commented=on  run=off  InputProcessing=Columns as channels (frame based)  reset_popup=None  directionMode=Each row  dimension=1  roiEnable=off  roiType=Rectangles  roiPortion=Entire ROI  roiOutput=Individual statistics for each ROI  roiFlag=off  roundingMode=Floor  overflowMode=off  outputDataTypeStr=Inherit: Same as accumulator  outputMin=[]  outputMax=[]  outputLastDataTypeStr=Inherit: Same as accumulator
  Mean 4 : dspstat3/Mean  Commented=on  run=off  InputProcessing=Columns as channels (frame based)  reset_popup=None  directionMode=Each row  dimension=1  roiEnable=off  roiType=Rectangles  roiPortion=Entire ROI  roiOutput=Individual statistics for each ROI  roiFlag=off  roundingMode=Floor  overflowMode=off  outputDataTypeStr=Inherit: Same as accumulator  outputMin=[]  outputMax=[]  outputLastDataTypeStr=Inherit: Same as accumulator
  "Product " : Product
  "Selector " : Selector  NumberOfDimensions=2  InputPortWidth=3  IndexOptions=Select all,Index vector (dialog)  Indices=[1 3],ones(20,1)  OutputSizes=1,1
  Out1 : Outport
  wires:
  Result from Channel Estimation/1 -> "Math Function "/1, Mean 1/1
  Mean 1/1 -> Math Function komplexe Konjugation/1
  Math Function komplexe Konjugation/1 -> Divide 2/1
  "Math Function "/1 -> Mean 2/1
  Mean 2/1 -> Divide 2/2
  Mean 3/1 -> Math Function komplexe Konjugation1/1
  Math Function 1/1 -> Mean 4/1
  Divide 2/1 -> "Selector "/1
  Data + Pilots/1 -> "Product "/2
  "Selector "/1 -> "Product "/1
  "Product "/1 -> Out1/1

== system Praktikum08Gruppe09/OFDM-Receiver /Channel Estimation ==
  note: We should divide recieved data to transmitted data
      | *remove 0, we can't divide to 0
  note: LTS(lange Trainingssequenz) [-26, 26] = {1, 1, -1, -1, 1, 1, -1, 1, -1, 1, 1, 1, 1, 1, 1, -1, -1, 1, 1, -1, 1, -1, 1, 1, 1, 1, 0, 1, -1, -1, 1, 1, -1, 1, -1, 1, -1, -1, -1, -1, -1, 1, 1, -1, -1, 1, -1, 1, -1, 1, 1, 1, 1}
  In1 : Inport
  "Divide " : Product  Inputs=*/
  "LTS [-26, 26]" : Constant  Value=complex([1, 1, -1, -1, 1, 1, -1, 1, -1, 1, 1, 1, 1, 1, 1, -1, -1, 1, 1, -1, 1, -1, 1, 1, 1, 1, 0, 1, -1, -1, 1, 1, -1, 1, -1, 1, -1, -1, -1, -1, -1, 1, 1, -1, -1, 1, -1, 1, -1, 1, 1, 1, 1])  VectorParams1D=off
  Matrix Concatenate 2 : Concatenate  Mode=Multidimensional array  ConcatenateDimension=2
  "Reshape " : Reshape  OutputDimensionality=Column vector (2-D)
  "Selector " : Selector  NumberOfDimensions=2  InputPortWidth=3  IndexOptions=Index vector (dialog),Select all  Indices=[1:26 28:53],1  OutputSizes=1,1
  Out1 : Outport
  wires:
  "LTS [-26, 26]"/1 -> "Reshape "/1
  "Reshape "/1 -> Matrix Concatenate 2/2, Matrix Concatenate 2/1
  Matrix Concatenate 2/1 -> "Selector "/1
  "Selector "/1 -> "Divide "/2
  In1/1 -> "Divide "/1
  "Divide "/1 -> Out1/1

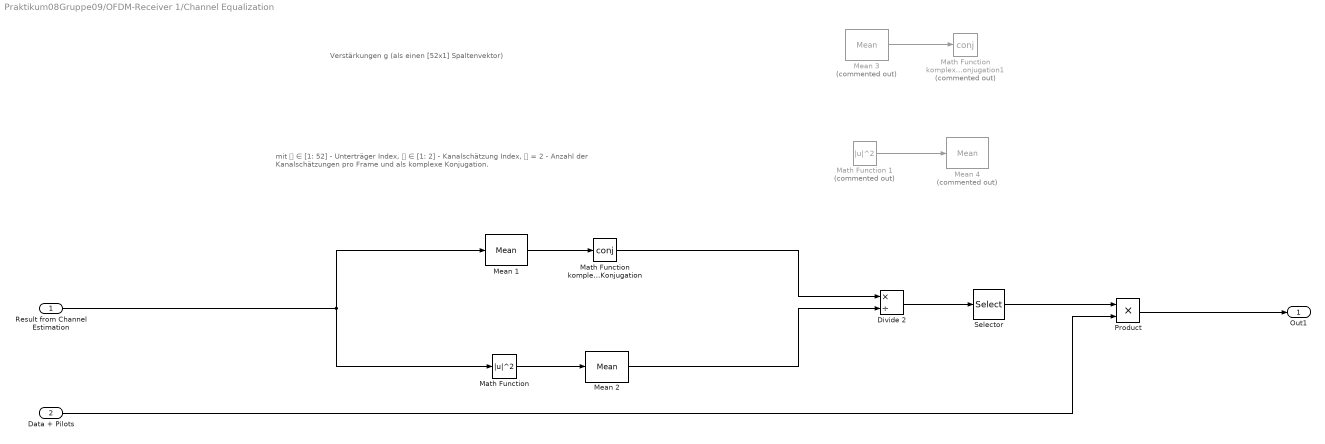
== system Praktikum08Gruppe09/OFDM-Receiver 1/Channel Equalization ==
  note: mit 𝑢 ∈ [1: 52] - Unterträger Index, 𝑛 ∈ [1: 2] - Kanalschätzung Index, 𝑁 = 2 - Anzahl der Kanalschätzungen pro Frame und als komplexe Konjugation.
  note: Verstärkungen g (als einen [52x1] Spaltenvektor)
  Result from Channel Estimation : Inport
  Data + Pilots : Inport  Port=2
  Divide 2 : Product  Inputs=*/
  "Math Function " : Math  Operator=magnitude^2
  Math Function 1 : Math  Commented=on  Operator=magnitude^2
  Math Function komplexe Konjugation : Math  Operator=conj  OutputSignalType=complex
  Math Function komplexe Konjugation1 : Math  Commented=on  Operator=conj  OutputSignalType=complex
  Mean 1 : dspstat3/Mean  run=off  InputProcessing=Columns as channels (frame based)  reset_popup=None  directionMode=Each row  dimension=1  roiEnable=off  roiType=Rectangles  roiPortion=Entire ROI  roiOutput=Individual statistics for each ROI  roiFlag=off  roundingMode=Floor  overflowMode=off  outputDataTypeStr=Inherit: Same as accumulator  outputMin=[]  outputMax=[]  outputLastDataTypeStr=Inherit: Same as accumulator
  Mean 2 : dspstat3/Mean  run=off  InputProcessing=Columns as channels (frame based)  reset_popup=None  directionMode=Each row  dimension=1  roiEnable=off  roiType=Rectangles  roiPortion=Entire ROI  roiOutput=Individual statistics for each ROI  roiFlag=off  roundingMode=Floor  overflowMode=off  outputDataTypeStr=Inherit: Same as accumulator  outputMin=[]  outputMax=[]  outputLastDataTypeStr=Inherit: Same as accumulator
  Mean 3 : dspstat3/Mean  Commented=on  run=off  InputProcessing=Columns as channels (frame based)  reset_popup=None  directionMode=Each row  dimension=1  roiEnable=off  roiType=Rectangles  roiPortion=Entire ROI  roiOutput=Individual statistics for each ROI  roiFlag=off  roundingMode=Floor  overflowMode=off  outputDataTypeStr=Inherit: Same as accumulator  outputMin=[]  outputMax=[]  outputLastDataTypeStr=Inherit: Same as accumulator
  Mean 4 : dspstat3/Mean  Commented=on  run=off  InputProcessing=Columns as channels (frame based)  reset_popup=None  directionMode=Each row  dimension=1  roiEnable=off  roiType=Rectangles  roiPortion=Entire ROI  roiOutput=Individual statistics for each ROI  roiFlag=off  roundingMode=Floor  overflowMode=off  outputDataTypeStr=Inherit: Same as accumulator  outputMin=[]  outputMax=[]  outputLastDataTypeStr=Inherit: Same as accumulator
  "Product " : Product
  "Selector " : Selector  NumberOfDimensions=2  InputPortWidth=3  IndexOptions=Select all,Index vector (dialog)  Indices=[1 3],ones(20,1)  OutputSizes=1,1
  Out1 : Outport
  wires:
  Result from Channel Estimation/1 -> "Math Function "/1, Mean 1/1
  Mean 1/1 -> Math Function komplexe Konjugation/1
  Math Function komplexe Konjugation/1 -> Divide 2/1
  "Math Function "/1 -> Mean 2/1
  Mean 2/1 -> Divide 2/2
  Mean 3/1 -> Math Function komplexe Konjugation1/1
  Math Function 1/1 -> Mean 4/1
  Divide 2/1 -> "Selector "/1
  Data + Pilots/1 -> "Product "/2
  "Selector "/1 -> "Product "/1
  "Product "/1 -> Out1/1

== system Praktikum08Gruppe09/OFDM-Receiver 1/Channel Estimation ==
  note: We should divide recieved data to transmitted data
      | *remove 0, we can't divide to 0
  note: LTS(lange Trainingssequenz) [-26, 26] = {1, 1, -1, -1, 1, 1, -1, 1, -1, 1, 1, 1, 1, 1, 1, -1, -1, 1, 1, -1, 1, -1, 1, 1, 1, 1, 0, 1, -1, -1, 1, 1, -1, 1, -1, 1, -1, -1, -1, -1, -1, 1, 1, -1, -1, 1, -1, 1, -1, 1, 1, 1, 1}
  In1 : Inport
  "Divide " : Product  Inputs=*/
  "LTS [-26, 26]" : Constant  Value=complex([1, 1, -1, -1, 1, 1, -1, 1, -1, 1, 1, 1, 1, 1, 1, -1, -1, 1, 1, -1, 1, -1, 1, 1, 1, 1, 0, 1, -1, -1, 1, 1, -1, 1, -1, 1, -1, -1, -1, -1, -1, 1, 1, -1, -1, 1, -1, 1, -1, 1, 1, 1, 1])  VectorParams1D=off
  Matrix Concatenate 2 : Concatenate  Mode=Multidimensional array  ConcatenateDimension=2
  "Reshape " : Reshape  OutputDimensionality=Column vector (2-D)
  "Selector " : Selector  NumberOfDimensions=2  InputPortWidth=3  IndexOptions=Index vector (dialog),Select all  Indices=[1:26 28:53],1  OutputSizes=1,1
  Out1 : Outport
  wires:
  "LTS [-26, 26]"/1 -> "Reshape "/1
  "Reshape "/1 -> Matrix Concatenate 2/2, Matrix Concatenate 2/1
  Matrix Concatenate 2/1 -> "Selector "/1
  "Selector "/1 -> "Divide "/2
  In1/1 -> "Divide "/1
  "Divide "/1 -> Out1/1
